simulink model "ai_optimal_path_depth_201009_3"  (R2020a)
settings: Solver=FixedStepDiscrete  StartTime=0.0  StopTime=inf  FixedStep=0.2  RelTol=1e-3  EnableMultiTasking=on
model workspace (MAT data in the model file):
  SL_ROS_VariableLengthArrays_MaxSizes : object (value not decoded)
undefined symbols (not defined in the file): Data, Data_SL_Info
libraries: robotlib x51
(part 2 of 2)

== matlab function ai_optimal_path_depth_201009_3/MATLAB Function2 ==
  data: odom_input input; point_cmd output; waypoint_pre input; waypoint_gen input; auto_flag output; waypoint_set output; Obstacle input; pos_init input
% % % function [point_cmd,auto_flag,waypoint_set,waypoint_pre_x,waypoint_pre_y,waypoint_pre_z] = gen_waypoint(pos_grid,waypoint_given,waypoint_gen,Obstacle)
function [point_cmd,auto_flag,waypoint_set]  = gen_waypoint(odom_input,waypoint_pre,waypoint_gen,Obstacle,pos_init)

persistent waypoint_flag autonomous_mode_flag waypoint_old

if isempty(waypoint_flag)
    waypoint_flag = zeros(10,1);
end
if isempty(autonomous_mode_flag)
    autonomous_mode_flag = 0;
end
if isempty(waypoint_old)
    waypoint_old = nan(20,3);
end

grid_size = 0.1;
replace_distance = 1;
odom = zeros(1,3);
odom(1,1) = odom_input.Pose.Pose.Position.X;
odom(1,2) = odom_input.Pose.Pose.Position.Y;
odom(1,3) = odom_input.Pose.Pose.Position.Z;
waypoint_pre_length = numel(waypoint_pre)/3;

if sum(waypoint_flag,'all') == waypoint_pre_length
    autonomous_mode_flag = 1;
end

waypoint_pre_x = waypoint_pre(:,1);
waypoint_pre_y = waypoint_pre(:,2);
waypoint_pre_z = waypoint_pre(:,3);
waypoint_pre_path_norm = inf(waypoint_pre_length,3);

waypoint_pre_path_norm(:,1) = waypoint_pre_x - odom(1);
waypoint_pre_path_norm(:,2) = waypoint_pre_y - odom(2);
waypoint_pre_path_norm(:,3) = waypoint_pre_z - odom(3);

K = inf(waypoint_pre_length,1);

for i = 1:waypoint_pre_length
    K(i) = norm(waypoint_pre_path_norm(i,:));
end

if (odom(1,1)^2+odom(1,2)^2) < 0.5
    point_cmd = [0, 0, odom(1,3)+0.2];  
else
    point_cmd = [odom(1,1) odom(1,2) odom(1,3)-10];  % Land (Maybe Hover)
end

waypoint_gen_sorted = nan(20,3);
waypoint_auto_set = nan(40,3);
waypoint_auto_set_sorted = nan(40,3);
waypoint_distance = nan(40,1);

for lll = 1:numel(waypoint_gen)/3
    if ~isnan(waypoint_gen(lll,1)) && ~isnan(waypoint_gen(lll,2)) && ~isnan(waypoint_gen(lll,3))
        if Obstacle(int8(waypoint_gen(lll,1)/grid_size+pos_init(1)),int8(waypoint_gen(lll,2)/grid_size+pos_init(2)),int8(waypoint_gen(lll,3)/grid_size+pos_init(3))) == 1
            waypoint_gen(lll,:)=nan(1,3);
        end
    end
end
for lll = 1:numel(waypoint_old)/3
    if ~isnan(waypoint_old(lll,1)) && ~isnan(waypoint_old(lll,2)) && ~isnan(waypoint_old(lll,3))
        if Obstacle(int8(waypoint_old(lll,1)/grid_size+pos_init(1)),int8(waypoint_old(lll,2)/grid_size+pos_init(2)),int8(waypoint_old(lll,3)/grid_size+pos_init(3))) == 1
            waypoint_old(lll,:)=nan(1,3);
        end
    end
end

if autonomous_mode_flag == 0
    for i = 1:waypoint_pre_length
        if waypoint_flag(i) == 0
            point_cmd = [waypoint_pre_x(i), waypoint_pre_y(i), waypoint_pre_z(i)];
            if K(i) < 0.2
                waypoint_flag(i) = 1;
            end
            break
        end
    end
elseif autonomous_mode_flag == 1
    waypoint_auto_old = waypoint_old;
    [~,waypoint_gen_index]=sort(waypoint_gen(:,1));
    for aaa = 1:length(waypoint_gen_index)
        waypoint_gen_sorted(aaa,:)=waypoint_gen(waypoint_gen_index(aaa),:);
    end
    waypoint_auto_new=waypoint_gen_sorted;
    if sum(isnan(waypoint_auto_old),'all')==numel(waypoint_auto_old)
        waypoint_auto_old = waypoint_auto_new;
    end
    
    num_nonnan_new = 0;
    num_nonnan_old = 0;
    for ttt = 1:numel(waypoint_auto_new)/3
        if ~isnan(waypoint_auto_new(ttt,1)) && ~isnan(waypoint_auto_new(ttt,2)) && ~isnan(waypoint_auto_new(ttt,3))
            num_nonnan_new = num_nonnan_new + 1;
        end
    end
    for sss = 1:numel(waypoint_auto_old)/3
        if ~isnan(waypoint_auto_old(sss,1)) && ~isnan(waypoint_auto_old(sss,2)) && ~isnan(waypoint_auto_old(sss,3))
            num_nonnan_old = num_nonnan_old + 1;
        end
    end
    
    if sum(isnan(waypoint_auto_old),'all')~=numel(waypoint_auto_old) && sum(isnan(waypoint_auto_new),'all')~=numel(waypoint_auto_new)
        for mmm = num_nonnan_new:-1:1
            changed_flag=0;
            for nnn = 1:num_nonnan_old
                if ((waypoint_auto_new(mmm,1)-waypoint_auto_old(nnn,1))^2+(waypoint_auto_new(mmm,2)-waypoint_auto_old(nnn,2))^2+(waypoint_auto_new(mmm,3)-waypoint_auto_old(nnn,3))^2)<replace_distance
                    waypoint_auto_old(nnn,:)=waypoint_auto_new(mmm,:);
                    changed_flag=1;
                end
            end
            if changed_flag == 1
                waypoint_auto_new(mmm,:)=nan(1,3);
            end
        end
        waypoint_auto_set_temp = cat(1,unique(waypoint_auto_old,'stable','rows'),waypoint_auto_new);
        
        
        for aaa = 1:numel(waypoint_auto_set_temp)/3
            waypoint_auto_set(aaa,:)=waypoint_auto_set_temp(aaa,:);
            waypoint_distance(aaa) = (((waypoint_auto_set(aaa,1)-odom(1))^2+(waypoint_auto_set(aaa,2)-odom(2))^2+(waypoint_auto_set(aaa,3)-odom(3))^2));
        end
        [~,waypoint_index]=sort(waypoint_distance);
        
        for aaa = 1:length(waypoint_index)
            waypoint_auto_set_sorted(aaa,:)=waypoint_auto_set(waypoint_index(aaa),:);
        end
        
        point_cmd = [waypoint_auto_set_sorted(1,1), waypoint_auto_set_sorted(1,2), waypoint_auto_set_sorted(1,3)];
        
        if sqrt((point_cmd(1)-odom(1)).^2+(point_cmd(2)-odom(2)).^2+(point_cmd(3)-odom(3)).^2) <= 0.2
            waypoint_auto_set_sorted = [waypoint_auto_set_sorted(2:end,:); nan(1,3)];
        end
        
        waypoint_old = waypoint_auto_set_sorted(1:20,:);
        
        
    else
        if ~isnan(waypoint_old(1,1)) && ~isnan(waypoint_old(1,2)) && ~isnan(waypoint_old(1,3))
            point_cmd = [waypoint_old(1,1), waypoint_old(1,2), waypoint_old(1,3)];
            
            if sqrt((point_cmd(1)-odom(1)).^2+(point_cmd(2)-odom(2)).^2+(point_cmd(3)-odom(3)).^2) <= 0.2
                waypoint_old = [waypoint_old(2:end,:); nan(1,3)];
            end
            
            
        else
            point_cmd = [odom(1,1) odom(1,2) odom(1,3)-10];  % Land (Maybe Hover)
        end
    end
end

% point_cmd = point_cmd_temp;


auto_flag = autonomous_mode_flag;
waypoint_set = waypoint_auto_set_sorted;
% % % % % % % %
% % % % % % % % persistent flag autonomous_mode_flag waypoint_old waypoint_pre
% % % % % % % %
% % % % % % % % if isempty(flag)
% % % % % % % %     flag = 1;
% % % % % % % % end
% % % % % % % % if isempty(autonomous_mode_flag)
% % % % % % % %     autonomous_mode_flag = 0;
% % % % % % % % %     autonomous_mode_flag = 1;
% % % % % % % % end
% % % % % % % % if isempty(waypoint_old)
% % % % % % % %     waypoint_old = nan(20,3);
% % % % % % % % end
% % % % % % % % % num_waypoint_given = numel(waypoint_given)/3;
% % % % % % % % num_waypoint_given = 1;
% % % % % % % % if isempty(waypoint_pre)
% % % % % % % %     waypoint_pre = nan(20,3);
% % % % % % % %     for aaa = 1:num_waypoint_given
% % % % % % % %         waypoint_pre(aaa,1)=waypoint_given(aaa,1);
% % % % % % % %         waypoint_pre(aaa,2)=waypoint_given(aaa,2);
% % % % % % % %         waypoint_pre(aaa,3)=waypoint_given(aaa,3);
% % % % % % % %     end
% % % % % % % % end
% % % % % % % %
% % % % % % % % pos_grid = int32(pos_grid);
% % % % % % % %
% % % % % % % % waypoint_pre_x = waypoint_pre(:,1);
% % % % % % % % waypoint_pre_y = waypoint_pre(:,2);
% % % % % % % % waypoint_pre_z = waypoint_pre(:,3);
% % % % % % % %
% % % % % % % % point_cmd_temp = int32([waypoint_pre_x(flag) waypoint_pre_y(flag) waypoint_pre_z(flag)]);
% % % % % % % % waypoint_gen_sorted = nan(20,3);
% % % % % % % % waypoint_auto_set = nan(40,3);
% % % % % % % % waypoint_auto_set_sorted = nan(40,3);
% % % % % % % % waypoint_distance = nan(40,1);
% % % % % % % %
% % % % % % % % for lll = 1:numel(waypoint_gen)/3
% % % % % % % %     if ~isnan(waypoint_gen(lll,1)) && ~isnan(waypoint_gen(lll,2)) && ~isnan(waypoint_gen(lll,3))
% % % % % % % %         if Obstacle(waypoint_gen(lll,1),waypoint_gen(lll,2),waypoint_gen(lll,3)) == 1
% % % % % % % %             waypoint_gen(lll,:)=nan(1,3);
% % % % % % % %         end
% % % % % % % %     end
% % % % % % % % end
% % % % % % % %
% % % % % % % %
% % % % % % % % if autonomous_mode_flag==0
% % % % % % % %     if abs(point_cmd_temp(1)-pos_grid(1)) <= 1 && abs(point_cmd_temp(2)-pos_grid(2)) <= 1 && abs(point_cmd_temp(3)-pos_grid(3)) <= 1
% % % % % % % %         flag = flag + 1;
% % % % % % % %
% % % % % % % %         %         if flag == numel(rmmissing(waypoint_pre))/3 + 1
% % % % % % % %         %             flag = numel(rmmissing(waypoint_pre))/3;
% % % % % % % % %         if flag == num_waypoint_given + 1
% % % % % % % %         if flag > num_waypoint_given
% % % % % % % %             flag = num_waypoint_given;
% % % % % % % %             autonomous_mode_flag = 1;
% % % % % % % %         end
% % % % % % % %     end
% % % % % % % %
% % % % % % % % elseif autonomous_mode_flag==1
% % % % % % % %     %     waypoint_auto_old = rmmissing(waypoint_old);
% % % % % % % %     %     waypoint_auto_new = rmmissing(waypoint_gen);
% % % % % % % %
% % % % % % % %
% % % % % % % %     waypoint_auto_old = waypoint_old;
% % % % % % % %     [~,waypoint_gen_index]=sort(waypoint_gen(:,1));
% % % % % % % %     for aaa = 1:length(waypoint_gen_index)
% % % % % % % %         waypoint_gen_sorted(aaa,:)=waypoint_gen(waypoint_gen_index(aaa),:);
% % % % % % % %     end
% % % % % % % %     waypoint_auto_new=waypoint_gen_sorted;
% % % % % % % % %     if isempty(waypoint_auto_old)
% % % % % % % %     if sum(isnan(waypoint_auto_old),'all')==numel(waypoint_auto_old)
% % % % % % % %         waypoint_auto_old = waypoint_auto_new;
% % % % % % % %     end
% % % % % % % %
% % % % % % % %     num_nonnan_new = 0;
% % % % % % % %     num_nonnan_old = 0;
% % % % % % % %     for ttt = 1:numel(waypoint_auto_new)/3
% % % % % % % %         if ~isnan(waypoint_auto_new(ttt,1)) && ~isnan(waypoint_auto_new(ttt,2)) && ~isnan(waypoint_auto_new(ttt,3))
% % % % % % % %             num_nonnan_new = num_nonnan_new + 1;
% % % % % % % %         end
% % % % % % % %     end
% % % % % % % %     for sss = 1:numel(waypoint_auto_old)/3
% % % % % % % %         if ~isnan(waypoint_auto_old(sss,1)) && ~isnan(waypoint_auto_old(sss,2)) && ~isnan(waypoint_auto_old(sss,3))
% % % % % % % %             num_nonnan_old = num_nonnan_old + 1;
% % % % % % % %         end
% % % % % % % %     end
% % % % % % % %
% % % % % % % % %     if ~isempty(waypoint_auto_old) && ~isempty(waypoint_auto_new)
% % % % % % % %     if sum(isnan(waypoint_auto_old),'all')~=numel(waypoint_auto_old) && sum(isnan(waypoint_auto_new),'all')~=numel(waypoint_auto_new)
% % % % % % % % %         for mmm = numel(waypoint_auto_new)/3:-1:1
% % % % % % % %         for mmm = num_nonnan_new:-1:1
% % % % % % % %             changed_flag=0;
% % % % % % % % %             for nnn = 1:numel(waypoint_auto_old)/3
% % % % % % % %             for nnn = 1:num_nonnan_old
% % % % % % % %                 if ((waypoint_auto_new(mmm,1)-waypoint_auto_old(nnn,1))^2+(waypoint_auto_new(mmm,2)-waypoint_auto_old(nnn,2))^2+(waypoint_auto_new(mmm,3)-waypoint_auto_old(nnn,3))^2)<100
% % % % % % % %                     waypoint_auto_old(nnn,:)=waypoint_auto_new(mmm,:);
% % % % % % % %                     changed_flag=1;
% % % % % % % %                 end
% % % % % % % %             end
% % % % % % % %             if changed_flag == 1
% % % % % % % %                 waypoint_auto_new(mmm,:)=nan(1,3);
% % % % % % % %             end
% % % % % % % %         end
% % % % % % % % %         waypoint_auto_set_temp = rmmissing(cat(1,unique(waypoint_auto_old,'stable','rows'),waypoint_auto_new));
% % % % % % % %         waypoint_auto_set_temp = cat(1,unique(waypoint_auto_old,'stable','rows'),waypoint_auto_new);
% % % % % % % %
% % % % % % % %
% % % % % % % %         for aaa = 1:numel(waypoint_auto_set_temp)/3
% % % % % % % %             waypoint_auto_set(aaa,:)=waypoint_auto_set_temp(aaa,:);
% % % % % % % %             waypoint_distance(aaa) = (((waypoint_auto_set(aaa,1)-pos_grid(1))^2+(waypoint_auto_set(aaa,2)-pos_grid(2))^2+(waypoint_auto_set(aaa,3)-pos_grid(3))^2));
% % % % % % % %         end
% % % % % % % %         [~,waypoint_index]=sort(waypoint_distance);
% % % % % % % %
% % % % % % % %         for aaa = 1:length(waypoint_index)
% % % % % % % %             waypoint_auto_set_sorted(aaa,:)=waypoint_auto_set(waypoint_index(aaa),:);
% % % % % % % %         end
% % % % % % % %
% % % % % % % %         point_cmd_temp = int32([waypoint_auto_set_sorted(1,1), waypoint_auto_set_sorted(1,2), waypoint_auto_set_sorted(1,3)]);
% % % % % % % %
% % % % % % % %         if abs(point_cmd_temp(1)-pos_grid(1)) <= 1 && abs(point_cmd_temp(2)-pos_grid(2)) <= 1 && abs(point_cmd_temp(3)-pos_grid(3)) <= 1
% % % % % % % %             waypoint_auto_set_sorted = [waypoint_auto_set_sorted(2:end,:); nan(1,3)];
% % % % % % % %         end
% % % % % % % %
% % % % % % % %         waypoint_old = waypoint_auto_set_sorted(1:20,:);
% % % % % % % %
% % % % % % % %
% % % % % % % %     else
% % % % % % % %         if ~isnan(waypoint_old(1,1)) && ~isnan(waypoint_old(1,2)) && ~isnan(waypoint_old(1,3))
% % % % % % % %             point_cmd_temp = int32([waypoint_old(1,1), waypoint_old(1,2), waypoint_old(1,3)]);
% % % % % % % %
% % % % % % % %             if abs(point_cmd_temp(1)-pos_grid(1)) <= 1 && abs(point_cmd_temp(2)-pos_grid(2)) <= 1 && abs(point_cmd_temp(3)-pos_grid(3)) <= 1
% % % % % % % %                 waypoint_old = [waypoint_old(2:end,:); nan(1,3)];
% % % % % % % %             end
% % % % % % % %
% % % % % % % %
% % % % % % % %         else
% % % % % % % %             point_cmd_temp = int32([pos_grid(1), pos_grid(2), pos_grid(3)]);
% % % % % % % %         end
% % % % % % % %     end
% % % % % % % % end
% % % % % % % %
% % % % % % % % point_cmd = point_cmd_temp;
% % % % % % % %
% % % % % % % %
% % % % % % % % auto_flag = autonomous_mode_flag;
% % % % % % % % waypoint_set = waypoint_auto_set_sorted;


end

== matlab function ai_optimal_path_depth_201009_3/MATLAB Function3 ==
  data: data input size=[1]; test output size=[1 512]; SL output
function [test,SL]   = func(data)

% test = single(nan(1,128));

test = single([data, nan(1,512-1)]);
% for i = 1:length(data)
%     test(i) = single(data(i));
% end

SL = uint32(length(data));


end

== matlab function ai_optimal_path_depth_201009_3/Empty Space Finding ==
  data: current_pos input; point input; distance input; bboxes_front_raw input; bboxes_back_raw input; bboxes_left_raw input; bboxes_right_raw input; emptypoint_front output; image_size input; image_grid input; emptypoint_back output; emptypoint_left output; emptypoint_right output; count output; obstacle_check output; emptypoint_front_temp output; emptypoint_back_temp output; emptypoint_left_temp output; emptypoint_right_temp output
function [emptypoint_front,emptypoint_back,emptypoint_left,emptypoint_right,count,obstacle_check,emptypoint_front_temp,emptypoint_back_temp,emptypoint_left_temp,emptypoint_right_temp] = fcn(current_pos,point,distance,bboxes_front_raw,bboxes_back_raw,bboxes_left_raw,bboxes_right_raw,image_size,image_grid)
% function [distance_ref_front,distance_ref_back,distance_ref_left,distance_ref_right] = fcn(point,I_front_rgb,I_back_rgb,I_left_rgb,I_right_rgb,bboxes_front_raw,bboxes_back_raw,bboxes_left_raw,bboxes_right_raw)



pos_x = current_pos.Pose.Pose.Position.X;
pos_y = current_pos.Pose.Pose.Position.Y;
pos_z = current_pos.Pose.Pose.Position.Z;

emptypoint_front = nan(5,6);
emptypoint_back = nan(5,6);
emptypoint_left = nan(5,6);
emptypoint_right = nan(5,6);
count = zeros(5,4);
obstacle_check = zeros(5,4);
thickness = distance/2;
% thickness = 2;
obstacle_safety = 0.5;
% obstacle_safety = 0.8;
obstacle_safety_height = 0.3;

bboxes_front = nan(5,4);
bboxes_back = nan(5,4);
bboxes_left = nan(5,4);
bboxes_right = nan(5,4);
for ttt = 1:4
    for sss = 1:5
        bboxes_front(sss,ttt) = int16(bboxes_front_raw(5*(ttt-1)+sss));
        bboxes_back(sss,ttt) = int16(bboxes_back_raw(5*(ttt-1)+sss));
        bboxes_left(sss,ttt) = int16(bboxes_left_raw(5*(ttt-1)+sss));
        bboxes_right(sss,ttt) = int16(bboxes_right_raw(5*(ttt-1)+sss));
    end
end
        
% distance_ref_front=[];
% distance_ref_back=[];
% distance_ref_left=[];
% distance_ref_right=[];

% % % % % % % % distance_ref_front=nan(5,1);
% % % % % % % % distance_ref_back=nan(5,1);
% % % % % % % % distance_ref_left=nan(5,1);
% % % % % % % % distance_ref_right=nan(5,1);
% % % % % % % % 
% % % % % % % % if ~sum(bboxes_front)==0
% % % % % % % %     for aaa = 1:numel(nonzeros(bboxes_front))/4
% % % % % % % %         if (bboxes_front(aaa,1)+bboxes_front(aaa,3)/2) >= (image_size)/2
% % % % % % % %             distance_ref_front(aaa) = bboxes_front(aaa,1)+bboxes_front(aaa,3);
% % % % % % % %         else
% % % % % % % %             distance_ref_front(aaa) = bboxes_front(aaa,1);
% % % % % % % %         end
% % % % % % % %     end
% % % % % % % %     distance_ref_front= -(distance_ref_front - (image_size)/2)*image_grid;           % 醫뚰몴媛?(m)
% % % % % % % % end
% % % % % % % % 
% % % % % % % % if ~sum(bboxes_back)==0
% % % % % % % %     for aaa = 1:numel(nonzeros(bboxes_back))/4
% % % % % % % %         if (bboxes_back(aaa,1)+bboxes_back(aaa,3)/2) >= (image_size)/2
% % % % % % % %             distance_ref_back(aaa) = bboxes_back(aaa,1)+bboxes_back(aaa,3);
% % % % % % % %         else
% % % % % % % %             distance_ref_back(aaa) = bboxes_back(aaa,1);
% % % % % % % %         end
% % % % % % % %     end
% % % % % % % %     distance_ref_back= -(distance_ref_back - (image_size)/2)*image_grid;              % 醫뚰몴媛?(m)
% % % % % % % % end
% % % % % % % % 
% % % % % % % % if ~sum(bboxes_left)==0
% % % % % % % %     for aaa = 1:numel(nonzeros(bboxes_left))/4
% % % % % % % %         if (bboxes_left(aaa,1)+bboxes_left(aaa,3)/2) >= (image_size)/2
% % % % % % % %             distance_ref_left(aaa) = bboxes_left(aaa,1)+bboxes_left(aaa,3);
% % % % % % % %         else
% % % % % % % %             distance_ref_left(aaa) = bboxes_left(aaa,1);
% % % % % % % %         end
% % % % % % % %     end
% % % % % % % %     distance_ref_left= (distance_ref_left - (image_size)/2)*image_grid;              % 醫뚰몴媛?(m)
% % % % % % % % end
% % % % % % % % 
% % % % % % % % % if ~isempty(bboxes_right)
% % % % % % % % if ~sum(bboxes_right)==0
% % % % % % % %     for aaa = 1:numel(nonzeros(bboxes_right))/4
% % % % % % % %         if (bboxes_right(aaa,1)+bboxes_right(aaa,3)/2) >= (image_size)/2
% % % % % % % %             distance_ref_right(aaa) = bboxes_right(aaa,1)+bboxes_right(aaa,3);
% % % % % % % %         else
% % % % % % % %             distance_ref_right(aaa) = bboxes_right(aaa,1);
% % % % % % % %         end
% % % % % % % %     end
% % % % % % % %     distance_ref_right= (distance_ref_right - (image_size)/2)*image_grid;            % 醫뚰몴媛?(m)
% % % % % % % % end
% % % % % % % % 
% % % % % % % % % scale = 5;
% % % % % % % % % scale = 20;
% % % % % % % % scale = 1/image_grid;
% % % % % % % % distance_fb_max=-ones(length(distance_ref_front),1)*image_grid*(image_size)/2;
% % % % % % % % distance_fb_min=ones(length(distance_ref_back),1)*image_grid*(image_size)/2;
% % % % % % % % distance_lr_max=-ones(length(distance_ref_left),1)*image_grid*(image_size)/2;
% % % % % % % % distance_lr_min=ones(length(distance_ref_right),1)*image_grid*(image_size)/2;
% % % % % % % % 
% % % % % % % % % distance_fb_max=ones(5,1)*distance;
% % % % % % % % % distance_fb_min=-ones(5,1)*distance;
% % % % % % % % % distance_lr_max=ones(5,1)*distance;
% % % % % % % % % distance_lr_min=-ones(5,1)*distance;
% % % % % % % %     
% % % % % % % % for bbb=1:length(point)
% % % % % % % %     %     if ~isempty(distance_ref_front)
% % % % % % % %     for aaa = 1:length(distance_ref_front)
% % % % % % % %         if ~isnan(distance_ref_front(aaa))
% % % % % % % %             if point(bbb,2)>=(distance_ref_front(aaa)-image_grid*scale) && point(bbb,2)<=(distance_ref_front(aaa)+image_grid*scale)
% % % % % % % %                 if point(bbb,1) > distance_fb_max(aaa)
% % % % % % % %                     distance_fb_max(aaa) = point(bbb,1);
% % % % % % % %                 end
% % % % % % % %             end
% % % % % % % %         end
% % % % % % % %     end
% % % % % % % %     %     if ~isempty(distance_ref_back)
% % % % % % % %     for aaa = 1:length(distance_ref_back)
% % % % % % % %         if ~isnan(distance_ref_back(aaa))
% % % % % % % %             if point(bbb,2)>=(distance_ref_back(aaa)-image_grid*scale) && point(bbb,2)<=(distance_ref_back(aaa)+image_grid*scale)
% % % % % % % %                 if point(bbb,1) < distance_fb_min(aaa)
% % % % % % % %                     distance_fb_min(aaa) = point(bbb,1);
% % % % % % % %                 end
% % % % % % % %             end
% % % % % % % %         end
% % % % % % % %     end
% % % % % % % %     %     if ~isempty(distance_ref_left)
% % % % % % % %     for aaa = 1:length(distance_ref_left)
% % % % % % % %         if ~isnan(distance_ref_left(aaa))
% % % % % % % %             if point(bbb,1)>=(distance_ref_left(aaa)-image_grid*scale) && point(bbb,1)<=(distance_ref_left(aaa)+image_grid*scale)
% % % % % % % %                 if point(bbb,2) > distance_lr_max(aaa)
% % % % % % % %                     distance_lr_max(aaa) = point(bbb,2);
% % % % % % % %                 end
% % % % % % % %             end
% % % % % % % %         end
% % % % % % % %     end
% % % % % % % %     %     if ~isempty(distance_ref_right)
% % % % % % % %     for aaa = 1:length(distance_ref_right)
% % % % % % % %         if ~isnan(distance_ref_right(aaa))
% % % % % % % %             if point(bbb,1)>=(distance_ref_right(aaa)-image_grid*scale) && point(bbb,1)<=(distance_ref_right(aaa)+image_grid*scale)
% % % % % % % %                 if point(bbb,2) < distance_lr_min(aaa)
% % % % % % % %                     distance_lr_min(aaa) = point(bbb,2);
% % % % % % % %                 end
% % % % % % % %             end
% % % % % % % %         end
% % % % % % % %     end
% % % % % % % % end
bboxes_transformed_front = -(double(bboxes_front)-[ones(5,1)*(image_size)/2, ones(5,1)*(image_size)/2, zeros(5,1), zeros(5,1)])*image_grid;
bboxes_transformed_back = -(double(bboxes_back)-[ones(5,1)*(image_size)/2, ones(5,1)*(image_size)/2, zeros(5,1), zeros(5,1)])*image_grid;
bboxes_transformed_left = (double(bboxes_left)-[ones(5,1)*(image_size)/2, ones(5,1)*(image_size)/2, zeros(5,1), zeros(5,1)]).*[ones(5,1), -ones(5,1), ones(5,1), -ones(5,1)]*image_grid;
bboxes_transformed_right = (double(bboxes_right)-[ones(5,1)*(image_size)/2, ones(5,1)*(image_size)/2, zeros(5,1), zeros(5,1)]).*[ones(5,1), -ones(5,1), ones(5,1), -ones(5,1)]*image_grid;

%(x,y,z,length,width,height)
% openpoint_front = [distance_fb_max-thickness/2,bboxes_transformed_front(:,1)+bboxes_transformed_front(:,3)/2,bboxes_transformed_front(:,2)+bboxes_transformed_front(:,4)/2,thickness*ones(length(distance_fb_max),1),abs(bboxes_transformed_front(:,3)),abs(bboxes_transformed_front(:,4))];                      
% openpoint_back = [distance_fb_min+thickness/2,bboxes_transformed_back(:,1)+bboxes_transformed_back(:,3)/2,bboxes_transformed_back(:,2)+bboxes_transformed_back(:,4)/2,thickness*ones(length(distance_fb_min),1),abs(bboxes_transformed_back(:,3)),abs(bboxes_transformed_back(:,4))];
% openpoint_left = [bboxes_transformed_left(:,1)+bboxes_transformed_left(:,3)/2 , distance_lr_max-thickness/2 , bboxes_transformed_left(:,2)+bboxes_transformed_left(:,4)/2,abs(bboxes_transformed_left(:,3)),thickness*ones(length(distance_lr_max),1),abs(bboxes_transformed_left(:,4))];
% openpoint_right = [bboxes_transformed_right(:,1)+bboxes_transformed_right(:,3)/2 , distance_lr_min+thickness/2 , bboxes_transformed_right(:,2)+bboxes_transformed_right(:,4)/2,abs(bboxes_transformed_right(:,3)),thickness*ones(length(distance_lr_min),1),abs(bboxes_transformed_right(:,4))];

for aaa = 1 : 5
%     if ~(distance_fb_max(aaa) == -image_grid*image_size/2)
    if ~isnan(bboxes_front(aaa,1))
%         emptypoint_front(aaa,:) = [distance_fb_max(aaa)-thickness/2 , bboxes_transformed_front(aaa,1)+bboxes_transformed_front(aaa,3)/2+pos_y , bboxes_transformed_front(aaa,2)+bboxes_transformed_front(aaa,4)/2+pos_z , thickness , abs(bboxes_transformed_front(aaa,3)) , abs(bboxes_transformed_front(aaa,4))];
        emptypoint_front(aaa,:) = [sqrt((distance-thickness/2).^2-( bboxes_transformed_front(aaa,1)+bboxes_transformed_front(aaa,3)/2).^2-( bboxes_transformed_front(aaa,2)+bboxes_transformed_front(aaa,4)/2).^2)+pos_x , bboxes_transformed_front(aaa,1)+bboxes_transformed_front(aaa,3)/2+pos_y , bboxes_transformed_front(aaa,2)+bboxes_transformed_front(aaa,4)/2+pos_z , thickness , abs(bboxes_transformed_front(aaa,3)) , abs(bboxes_transformed_front(aaa,4))];
    end
%     if ~(distance_fb_min(aaa) == image_grid*image_size/2)
    if ~isnan(bboxes_back(aaa,1))
%         emptypoint_back(aaa,:) = [distance_fb_min(aaa)+thickness/2 , bboxes_transformed_back(aaa,1)+bboxes_transformed_back(aaa,3)/2+pos_y , bboxes_transformed_back(aaa,2)+bboxes_transformed_back(aaa,4)/2+pos_z , thickness , abs(bboxes_transformed_back(aaa,3)) , abs(bboxes_transformed_back(aaa,4))];
        emptypoint_back(aaa,:) = [-sqrt((distance-thickness/2).^2-(bboxes_transformed_back(aaa,1)+bboxes_transformed_back(aaa,3)/2).^2-(bboxes_transformed_back(aaa,2)+bboxes_transformed_back(aaa,4)/2).^2)+pos_x , bboxes_transformed_back(aaa,1)+bboxes_transformed_back(aaa,3)/2+pos_y , bboxes_transformed_back(aaa,2)+bboxes_transformed_back(aaa,4)/2+pos_z , thickness , abs(bboxes_transformed_back(aaa,3)) , abs(bboxes_transformed_back(aaa,4))];
    end
%     if ~(distance_lr_max(aaa) == -image_grid*image_size/2)
    if ~isnan(bboxes_left(aaa,1))
%         emptypoint_left(aaa,:) = [bboxes_transformed_left(aaa,1)+bboxes_transformed_left(aaa,3)/2+pos_x , distance_lr_max(aaa)-thickness/2 , bboxes_transformed_left(aaa,2)+bboxes_transformed_left(aaa,4)/2+pos_z , abs(bboxes_transformed_left(aaa,3)) , thickness , abs(bboxes_transformed_left(aaa,4))];
        emptypoint_left(aaa,:) = [bboxes_transformed_left(aaa,1)+bboxes_transformed_left(aaa,3)/2+pos_x , sqrt((distance-thickness/2).^2-(bboxes_transformed_left(aaa,1)+bboxes_transformed_left(aaa,3)/2).^2-(bboxes_transformed_left(aaa,2)+bboxes_transformed_left(aaa,4)/2).^2)+pos_y , bboxes_transformed_left(aaa,2)+bboxes_transformed_left(aaa,4)/2+pos_z , abs(bboxes_transformed_left(aaa,3)) , thickness , abs(bboxes_transformed_left(aaa,4))];
    end
%     if ~(distance_lr_min(aaa) == image_grid*image_size/2)
    if ~isnan(bboxes_right(aaa,1))
%         emptypoint_right(aaa,:) = [bboxes_transformed_right(aaa,1)+bboxes_transformed_right(aaa,3)/2+pos_x , distance_lr_min(aaa)+thickness/2 , bboxes_transformed_right(aaa,2)+bboxes_transformed_right(aaa,4)/2+pos_z , abs(bboxes_transformed_right(aaa,3)) , thickness , abs(bboxes_transformed_right(aaa,4))];
        emptypoint_right(aaa,:) = [bboxes_transformed_right(aaa,1)+bboxes_transformed_right(aaa,3)/2+pos_x , -sqrt((distance-thickness/2).^2-(bboxes_transformed_right(aaa,1)+bboxes_transformed_right(aaa,3)/2).^2-(bboxes_transformed_right(aaa,2)+bboxes_transformed_right(aaa,4)/2).^2)+pos_y , bboxes_transformed_right(aaa,2)+bboxes_transformed_right(aaa,4)/2+pos_z , abs(bboxes_transformed_right(aaa,3)) , thickness , abs(bboxes_transformed_right(aaa,4))];
    end
end

emptypoint_front_temp = emptypoint_front;
emptypoint_back_temp = emptypoint_back;
emptypoint_left_temp = emptypoint_left;
emptypoint_right_temp = emptypoint_right;

for aaa = 1:5
    count_front = 0;
    count_back = 0;
    count_left = 0;
    count_right = 0;
    obstacle_check_front = 0;
    obstacle_check_back = 0;
    obstacle_check_left = 0;
    obstacle_check_right = 0;
    for bbb = 1:length(point)
%         if ((point(bbb,1) > emptypoint_front(aaa,1)-thickness/10) && (point(bbb,1) < emptypoint_front(aaa,1)+thickness/10)) && (point(bbb,2) > emptypoint_front(aaa,2)-thickness/10) && (point(bbb,2) < emptypoint_front(aaa,2)+thickness/10)
        if ((point(bbb,1) > emptypoint_front(aaa,1)-obstacle_safety) && (point(bbb,1) < emptypoint_front(aaa,1)+obstacle_safety)) && (point(bbb,2) > emptypoint_front(aaa,2)-obstacle_safety) && (point(bbb,2) < emptypoint_front(aaa,2)+obstacle_safety)
            count_front = count_front+1;
        end
%         if ((point(bbb,1) > emptypoint_back(aaa,1)-thickness/10) && (point(bbb,1) < emptypoint_back(aaa,1)+thickness/10)) && (point(bbb,2) > emptypoint_back(aaa,2)-thickness/10) && (point(bbb,2) < emptypoint_back(aaa,2)+thickness/10)
        if ((point(bbb,1) > emptypoint_back(aaa,1)-obstacle_safety) && (point(bbb,1) < emptypoint_back(aaa,1)+obstacle_safety)) && (point(bbb,2) > emptypoint_back(aaa,2)-obstacle_safety) && (point(bbb,2) < emptypoint_back(aaa,2)+obstacle_safety)
            count_back = count_back+1;
        end
%         if ((point(bbb,1) > emptypoint_left(aaa,1)-thickness/10) && (point(bbb,1) < emptypoint_left(aaa,1)+thickness/10)) && (point(bbb,2) > emptypoint_left(aaa,2)-thickness/10) && (point(bbb,2) < emptypoint_left(aaa,2)+thickness/10)
        if ((point(bbb,1) > emptypoint_left(aaa,1)-obstacle_safety) && (point(bbb,1) < emptypoint_left(aaa,1)+obstacle_safety)) && (point(bbb,2) > emptypoint_left(aaa,2)-obstacle_safety) && (point(bbb,2) < emptypoint_left(aaa,2)+obstacle_safety)
            count_left = count_left+1;
        end
%         if ((point(bbb,1) > emptypoint_right(aaa,1)-thickness/10) && (point(bbb,1) < emptypoint_right(aaa,1)+thickness/10)) && (point(bbb,2) > emptypoint_right(aaa,2)-thickness/10) && (point(bbb,2) < emptypoint_right(aaa,2)+thickness/10)
        if ((point(bbb,1) > emptypoint_right(aaa,1)-obstacle_safety) && (point(bbb,1) < emptypoint_right(aaa,1)+obstacle_safety)) && (point(bbb,2) > emptypoint_right(aaa,2)-obstacle_safety) && (point(bbb,2) < emptypoint_right(aaa,2)+obstacle_safety)
            count_right= count_right+1;
        end
        
        if ((point(bbb,1) > emptypoint_front(aaa,1)-obstacle_safety) && (point(bbb,1) < emptypoint_front(aaa,1)+obstacle_safety)) && ((point(bbb,2) > emptypoint_front(aaa,2)-obstacle_safety) && (point(bbb,2) < emptypoint_front(aaa,2)+obstacle_safety)) && ((point(bbb,3) > emptypoint_front(aaa,3)-obstacle_safety_height) && (point(bbb,3) < emptypoint_front(aaa,3)+obstacle_safety_height))
            obstacle_check_front = obstacle_check_front+1;
        end
        if ((point(bbb,1) > emptypoint_back(aaa,1)-obstacle_safety) && (point(bbb,1) < emptypoint_back(aaa,1)+obstacle_safety)) && ((point(bbb,2) > emptypoint_back(aaa,2)-obstacle_safety) && (point(bbb,2) < emptypoint_back(aaa,2)+obstacle_safety)) && ((point(bbb,3) > emptypoint_back(aaa,3)-obstacle_safety_height) && (point(bbb,3) < emptypoint_back(aaa,3)+obstacle_safety_height))
            obstacle_check_back = obstacle_check_back+1;
        end
        if ((point(bbb,1) > emptypoint_left(aaa,1)-obstacle_safety) && (point(bbb,1) < emptypoint_left(aaa,1)+obstacle_safety)) && ((point(bbb,2) > emptypoint_left(aaa,2)-obstacle_safety) && (point(bbb,2) < emptypoint_left(aaa,2)+obstacle_safety)) && ((point(bbb,3) > emptypoint_left(aaa,3)-obstacle_safety_height) && (point(bbb,3) < emptypoint_left(aaa,3)+obstacle_safety_height))
            obstacle_check_left = obstacle_check_left+1;
        end
        if ((point(bbb,1) > emptypoint_right(aaa,1)-obstacle_safety) && (point(bbb,1) < emptypoint_right(aaa,1)+obstacle_safety)) && ((point(bbb,2) > emptypoint_right(aaa,2)-obstacle_safety) && (point(bbb,2) < emptypoint_right(aaa,2)+obstacle_safety)) && ((point(bbb,3) > emptypoint_right(aaa,3)-obstacle_safety_height) && (point(bbb,3) < emptypoint_right(aaa,3)+obstacle_safety_height))
            obstacle_check_right= obstacle_check_right+1;
        end
        
    end
    %유효성 체크
    count(aaa,:) = [count_front, count_back, count_left, count_right];
    obstacle_check(aaa,:) = [obstacle_check_front, obstacle_check_back, obstacle_check_left, obstacle_check_right];
    if count_front < 5 || obstacle_check_front > 0
%     if obstacle_check_front > 0
        emptypoint_front(aaa,:) = nan(1,6);
    end
    if count_back< 5 || obstacle_check_back > 0
%     if obstacle_check_back > 0
        emptypoint_back(aaa,:) = nan(1,6);
    end
    if count_left< 5 || obstacle_check_left > 0
%     if obstacle_check_left > 0
        emptypoint_left(aaa,:) = nan(1,6);
    end
    if count_right< 5 || obstacle_check_right > 0
%     if obstacle_check_right > 0
        emptypoint_right(aaa,:) = nan(1,6);
    end
end

== matlab function ai_optimal_path_depth_201009_3/Waypoint Generation ==
  data: pos_cur input; distance input; waypoint_gen output; emptypoint_front input; emptypoint_back input; emptypoint_left input; emptypoint_right input; exploration output
function [waypoint_gen,exploration] = fcn(pos_cur,distance,emptypoint_front,emptypoint_back,emptypoint_left,emptypoint_right)

persistent explor_grid

if isempty(explor_grid)
    explor_grid = zeros(50,50,10);
end

pos_x = pos_cur.Pose.Pose.Position.X;
pos_y = pos_cur.Pose.Pose.Position.Y;
pos_z = pos_cur.Pose.Pose.Position.Z;

% grid_explor_size = 4;
grid_explor_size = distance/2;
% grid_explor_size = distance/4;
explor_map_init = [25, 25, 5];
% pos_explor_grid = int32([pos_x/grid_explor_size+explor_map_init(1), pos_y/grid_explor_size+explor_map_init(2) , pos_z/grid_explor_size+explor_map_init(3)]);

pos_explor_grid1 = int32([(pos_x+grid_explor_size/2)/grid_explor_size+explor_map_init(1), (pos_y+grid_explor_size/2)/grid_explor_size+explor_map_init(2) , (pos_z+grid_explor_size/2)/grid_explor_size+explor_map_init(3)]);
pos_explor_grid2 = int32([(pos_x+grid_explor_size/2)/grid_explor_size+explor_map_init(1), (pos_y-grid_explor_size/2)/grid_explor_size+explor_map_init(2) , (pos_z+grid_explor_size/2)/grid_explor_size+explor_map_init(3)]);
pos_explor_grid3 = int32([(pos_x-grid_explor_size/2)/grid_explor_size+explor_map_init(1), (pos_y+grid_explor_size/2)/grid_explor_size+explor_map_init(2) , (pos_z+grid_explor_size/2)/grid_explor_size+explor_map_init(3)]);
pos_explor_grid4 = int32([(pos_x-grid_explor_size/2)/grid_explor_size+explor_map_init(1), (pos_y-grid_explor_size/2)/grid_explor_size+explor_map_init(2) , (pos_z+grid_explor_size/2)/grid_explor_size+explor_map_init(3)]);
pos_explor_grid5 = int32([(pos_x+grid_explor_size/2)/grid_explor_size+explor_map_init(1), (pos_y+grid_explor_size/2)/grid_explor_size+explor_map_init(2) , (pos_z-grid_explor_size/2)/grid_explor_size+explor_map_init(3)]);
pos_explor_grid6 = int32([(pos_x+grid_explor_size/2)/grid_explor_size+explor_map_init(1), (pos_y-grid_explor_size/2)/grid_explor_size+explor_map_init(2) , (pos_z-grid_explor_size/2)/grid_explor_size+explor_map_init(3)]);
pos_explor_grid7 = int32([(pos_x-grid_explor_size/2)/grid_explor_size+explor_map_init(1), (pos_y+grid_explor_size/2)/grid_explor_size+explor_map_init(2) , (pos_z-grid_explor_size/2)/grid_explor_size+explor_map_init(3)]);
pos_explor_grid8 = int32([(pos_x-grid_explor_size/2)/grid_explor_size+explor_map_init(1), (pos_y-grid_explor_size/2)/grid_explor_size+explor_map_init(2) , (pos_z-grid_explor_size/2)/grid_explor_size+explor_map_init(3)]);
% explor_grid(pos_explor_grid(1),pos_explor_grid(2),pos_explor_grid(3))=1;

explor_grid(pos_explor_grid1(1),pos_explor_grid1(2),pos_explor_grid1(3))=1;
explor_grid(pos_explor_grid2(1),pos_explor_grid2(2),pos_explor_grid2(3))=1;
explor_grid(pos_explor_grid3(1),pos_explor_grid3(2),pos_explor_grid3(3))=1;
explor_grid(pos_explor_grid4(1),pos_explor_grid4(2),pos_explor_grid4(3))=1;
explor_grid(pos_explor_grid5(1),pos_explor_grid5(2),pos_explor_grid5(3))=1;
explor_grid(pos_explor_grid6(1),pos_explor_grid6(2),pos_explor_grid6(3))=1;
explor_grid(pos_explor_grid7(1),pos_explor_grid7(2),pos_explor_grid7(3))=1;
explor_grid(pos_explor_grid8(1),pos_explor_grid8(2),pos_explor_grid8(3))=1;

for abc=1:numel(emptypoint_front)/6
    if ~isnan(emptypoint_front(abc,1)) && ~isnan(emptypoint_front(abc,2)) && ~isnan(emptypoint_front(abc,3))
        if explor_grid(int16(emptypoint_front(abc,1)/grid_explor_size+explor_map_init(1)),int16(emptypoint_front(abc,2)/grid_explor_size+explor_map_init(2)),int16(emptypoint_front(abc,3)/grid_explor_size+explor_map_init(3))) == 1
            emptypoint_front(abc,:) = nan(1,6);
        end
    end
end
for abc=1:numel(emptypoint_back)/6
    if ~isnan(emptypoint_back(abc,1)) && ~isnan(emptypoint_back(abc,2)) && ~isnan(emptypoint_back(abc,3))
        if explor_grid(int16(emptypoint_back(abc,1)/grid_explor_size+explor_map_init(1)),int16(emptypoint_back(abc,2)/grid_explor_size+explor_map_init(2)),int16(emptypoint_back(abc,3)/grid_explor_size+explor_map_init(3))) == 1
            emptypoint_back(abc,:) = nan(1,6);
        end
    end
end
for abc=1:numel(emptypoint_left)/6
    if ~isnan(emptypoint_left(abc,1)) && ~isnan(emptypoint_left(abc,2)) && ~isnan(emptypoint_left(abc,3))
        if explor_grid(int16(emptypoint_left(abc,1)/grid_explor_size+explor_map_init(1)),int16(emptypoint_left(abc,2)/grid_explor_size+explor_map_init(2)),int16(emptypoint_left(abc,3)/grid_explor_size+explor_map_init(3))) == 1
            emptypoint_left(abc,:) = nan(1,6);
        end
    end
end
for abc=1:numel(emptypoint_right)/6
    if ~isnan(emptypoint_right(abc,1)) && ~isnan(emptypoint_right(abc,2)) && ~isnan(emptypoint_right(abc,3))
        if explor_grid(int16(emptypoint_right(abc,1)/grid_explor_size+explor_map_init(1)),int16(emptypoint_right(abc,2)/grid_explor_size+explor_map_init(2)),int16(emptypoint_right(abc,3)/grid_explor_size+explor_map_init(3))) == 1
            emptypoint_right(abc,:) = nan(1,6);
        end
    end
end



waypoint_gen_front = nan(5,3);
waypoint_gen_back = nan(5,3);
waypoint_gen_left = nan(5,3);
waypoint_gen_right = nan(5,3);

for aaa = 1:5
        waypoint_gen_front(aaa,:) = [emptypoint_front(aaa,1), emptypoint_front(aaa,2), emptypoint_front(aaa,3)];
        waypoint_gen_back(aaa,:) = [emptypoint_back(aaa,1), emptypoint_back(aaa,2), emptypoint_back(aaa,3)];
        waypoint_gen_left(aaa,:) = [emptypoint_left(aaa,1), emptypoint_left(aaa,2), emptypoint_left(aaa,3)];
        waypoint_gen_right(aaa,:) = [emptypoint_right(aaa,1), emptypoint_right(aaa,2), emptypoint_right(aaa,3)];
end


exploration =explor_grid;
waypoint_gen = [waypoint_gen_front;waypoint_gen_back;waypoint_gen_left;waypoint_gen_right];

%%%%%%%%%%%%%%%%%%%%%%%%%%%%%%%%%%%% for back safety
for lll = 1:numel(waypoint_gen)/3
    if waypoint_gen(lll,1)<-0.5
        waypoint_gen(lll,:) = nan(1,3);
    end
end

== matlab function ai_optimal_path_depth_201009_3/MATLAB Function5 ==
  data: data input size=[40 3]; test output size=[1 512]; SL output
function [test,SL]   = func(data)

% test = single(nan(1,128));

test = single([data(:,1)', nan(1,512-40)]);
% for i = 1:length(data)
%     test(i) = single(data(i));
% end

SL = uint32(length(data(:,1)));


end
